simulink model "TRAMI_DCT_AT"  (R2018b)
settings: Solver=FixedStepDiscrete  StartTime=0.0  StopTime=88  FixedStep=10e-3  RelTol=1e-3  EnableMultiTasking=on
undefined symbols (not defined in the file): CONST_AP_GEAR_SUB_NEWTRAL, CONST_AP_IDLE_SPEED_CONT, CONST_AP_LOAD_SFT, CONST_AP_LOAD_SFT_HYS, CONST_CAR_WEIGHT, CONST_CL_NUM, CONST_F_DOWN_SYNCHRO, CONST_F_SYNCHRO, CONST_F_UP_SYNCHRO, CONST_FGR, CONST_I_FlYWHEEL, CONST_INATIA_CLANK, CONST_R_SHIFT_END_CD, CONST_R_SHIFT_END_EG, CONST_R_SHIFT_END_TD, CONST_R_SHIFT_END_UP, CONST_R_SYNCHRO_ENGAGE, CONST_R_TIRE, CONST_RATIO_TQ_REDUCTION, CONST_SKIP_SHIFT_MAX, CONST_SYN_NUM, CONST_T_SFT_END_EN, CONST_T_SFT_END_JUDGE, CONST_T_SFT_END_MAX, CONST_T_SFT_END_MIN, CONST_T_SHIFT_WAIT, CONST_T_TQ_PHASE_CD, CONST_T_TQ_PHASE_ND, CONST_T_TQ_PHASE_NR, CONST_T_TQ_PHASE_TD, CONST_T_TQ_PHASE_UP, CONST_TQ_CREEP_CONT, CONST_TQ_ENGAGE_CL_MARGIN, CONST_TQ_ENGAGE_CL_MIN, CONST_TQ_INATIA_TD_SHIFT, CONST_TQ_LOAD_SFT, CONST_TQ_LOAD_SFT_HYS, CONST_TQ_ND_ENGAGE, CONST_TQ_NR_ENGAGE, CONST_TQ_TQPHASE_MIN, CONST_V_IDLE_SPEED_CONT, Eng, FALSE, GrNP, GrRev, LoopTime, MAT_CL_ENGAGE, MAT_CL_SHARE_RATE, MAT_I_ACTUATOR, MAT_SYNCHRO_COM, MAT_T_GEAR_SUB_NEWTRAL, MAT_TRANS_MGR, MaxCL, Nm, PI, Shift_CD, Shift_ND, Shift_NR, Shift_TD, Shift_Up ... (+168)
libraries: simulink x26
(part 1 of 6)
settings Model: Creator=yuto-n  LastModifiedBy=yuto-n
settings DataIOCC: SaveFormat=Array  SaveOutput=off  SignalLogging=off  DSMLogging=off  SaveTime=off
settings OptimizationCC: LifeSpan=inf
settings DebuggingCC: MultiTaskRateTransMsg=warning  ParameterPrecisionLossMsg=none
settings ModelReferenceCC: PropagateSignalLabelsOutOfModel=off

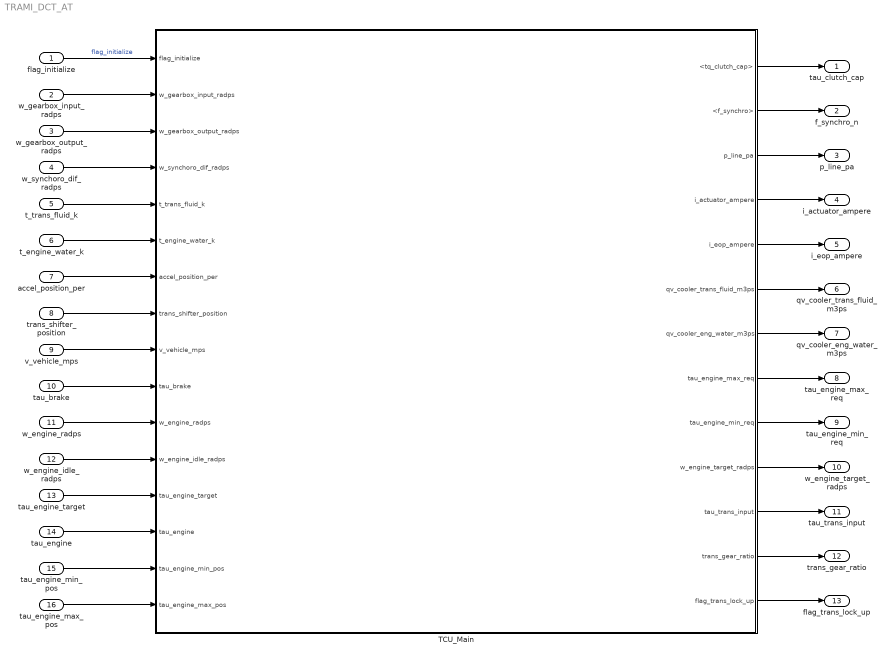
== system TRAMI_DCT_AT ==
  flag_initialize : Inport  OutDataTypeStr=boolean
      settings: AttributesFormatString=イニシャライズ要求
  w_gearbox_input_radps : Inport  Port=2  OutDataTypeStr=single
      settings: AttributesFormatString=Gearbox input speed[rad/s]
  w_gearbox_output_radps : Inport  Port=3  OutDataTypeStr=single
      settings: AttributesFormatString=Gearbox output speed[rad/s]
  w_synchoro_dif_radps : Inport  Port=4  OutDataTypeStr=single  PortDimensions=MaxSyn
      settings: AttributesFormatString=各シンクロ差回転[rad/s]
  t_trans_fluid_k : Inport  Port=5  OutDataTypeStr=single
      settings: AttributesFormatString=トランスミッション油温[K]
  t_engine_water_k : Inport  Port=6  OutDataTypeStr=single
      settings: AttributesFormatString=Eng.冷却水温[K]
  accel_position_per : Inport  Port=7  OutDataTypeStr=single
      settings: AttributesFormatString=アクセル開度[%]
  trans_shifter_position : Inport  Port=8  OutDataTypeStr=int16
      settings: AttributesFormatString=シフト位置 Rev=-1; N=0 ; D=1
  v_vehicle_mps : Inport  Port=9  OutDataTypeStr=single
      settings: AttributesFormatString=車速[m/s]
  tau_brake : Inport  Port=10  OutDataTypeStr=single
      settings: AttributesFormatString=ブレーキトルク[Nm]
  w_engine_radps : Inport  Port=11  OutDataTypeStr=single
      settings: AttributesFormatString=Engine回転[rad/s]
  w_engine_idle_radps : Inport  Port=12  OutDataTypeStr=single
      settings: AttributesFormatString=Engineアイドル回転[rad/s]
  tau_engine_target : Inport  Port=13  OutDataTypeStr=single
      settings: AttributesFormatString=Engine 目標トルク[Nm]
  tau_engine : Inport  Port=14  OutDataTypeStr=single
      settings: AttributesFormatString=Engine トルク[Nm]
  tau_engine_min_pos : Inport  Port=15  OutDataTypeStr=single
      settings: AttributesFormatString=Eng.出力可能最小トルク[Nm]
  tau_engine_max_pos : Inport  Port=16  OutDataTypeStr=single
      settings: AttributesFormatString=Eng.出力可能最小トルク[Nm]
  TCU_Main : Subsystem  TreatAsAtomicUnit=on  SystemSampleTime=0.01
      settings: AttributesFormatString=Transmission制御
  tau_clutch_cap : Outport  OutDataTypeStr=single
      settings: AttributesFormatString=各クラッチのトルク容量[Nm]
  f_synchro_n : Outport  Port=2  OutDataTypeStr=single
      settings: AttributesFormatString=各シンクロの操作力[N]
  p_line_pa : Outport  Port=3  OutDataTypeStr=single
      settings: AttributesFormatString=ライン圧[Pa]
  i_actuator_ampere : Outport  Port=4  OutDataTypeStr=single
      settings: AttributesFormatString=アクチュエータ電流[A]
  i_eop_ampere : Outport  Port=5  OutDataTypeStr=single
      settings: AttributesFormatString=電動オイルポンプ電流[A]
  qv_cooler_trans_fluid_m3ps : Outport  Port=6  OutDataTypeStr=single
      settings: AttributesFormatString=クーラーのATF流量[m3/s]
  qv_cooler_eng_water_m3ps : Outport  Port=7  OutDataTypeStr=single
      settings: AttributesFormatString=クーラーの冷却水流量[m3/s]
  tau_engine_max_req : Outport  Port=8  OutDataTypeStr=single
      settings: AttributesFormatString=エンジントルクリダクション要求[Nm]
  tau_engine_min_req : Outport  Port=9  OutDataTypeStr=single
      settings: AttributesFormatString=エンジントルクアップ要求[Nm]
  w_engine_target_radps : Outport  Port=10  OutDataTypeStr=single
      settings: AttributesFormatString=エンジン回転要求値[rad/s]
  tau_trans_input : Outport  Port=11  OutDataTypeStr=single
      settings: AttributesFormatString=トランスミッション入力軸トルク[Nm]
  trans_gear_ratio : Outport  Port=12  OutDataTypeStr=single
      settings: AttributesFormatString=ギヤ比
  flag_trans_lock_up : Outport  Port=13  OutDataTypeStr=boolean
      settings: AttributesFormatString=ロックアップ判定
  wires:
  tau_engine_max_pos/1 -> TCU_Main/16(tau_engine_max_pos)
  w_engine_idle_radps/1 -> TCU_Main/12(w_engine_idle_radps)
  accel_position_per/1 -> TCU_Main/7(accel_position_per)
  w_engine_radps/1 -> TCU_Main/11(w_engine_radps)
  tau_brake/1 -> TCU_Main/10(tau_brake)
  trans_shifter_position/1 -> TCU_Main/8(trans_shifter_position)
  t_engine_water_k/1 -> TCU_Main/6(t_engine_water_k)
  flag_initialize/1 -> TCU_Main/1(flag_initialize)  "flag_initialize"
  w_gearbox_input_radps/1 -> TCU_Main/2(w_gearbox_input_radps)
  TCU_Main/2(<f_synchro>) -> f_synchro_n/1
  TCU_Main/1(<tq_clutch_cap>) -> tau_clutch_cap/1
  tau_engine_target/1 -> TCU_Main/13(tau_engine_target)
  TCU_Main/11(tau_trans_input) -> tau_trans_input/1
  w_synchoro_dif_radps/1 -> TCU_Main/4(w_synchoro_dif_radps)
  tau_engine_min_pos/1 -> TCU_Main/15(tau_engine_min_pos)
  TCU_Main/9(tau_engine_min_req) -> tau_engine_min_req/1
  w_gearbox_output_radps/1 -> TCU_Main/3(w_gearbox_output_radps)
  TCU_Main/13(flag_trans_lock_up) -> flag_trans_lock_up/1
  TCU_Main/12(trans_gear_ratio) -> trans_gear_ratio/1
  tau_engine/1 -> TCU_Main/14(tau_engine)
  TCU_Main/4(i_actuator_ampere) -> i_actuator_ampere/1
  t_trans_fluid_k/1 -> TCU_Main/5(t_trans_fluid_k)
  v_vehicle_mps/1 -> TCU_Main/9(v_vehicle_mps)
  TCU_Main/10(w_engine_target_radps) -> w_engine_target_radps/1
  TCU_Main/3(p_line_pa) -> p_line_pa/1
  TCU_Main/6(qv_cooler_trans_fluid_m3ps) -> qv_cooler_trans_fluid_m3ps/1
  TCU_Main/7(qv_cooler_eng_water_m3ps) -> qv_cooler_eng_water_m3ps/1
  TCU_Main/5(i_eop_ampere) -> i_eop_ampere/1
  TCU_Main/8(tau_engine_max_req) -> tau_engine_max_req/1

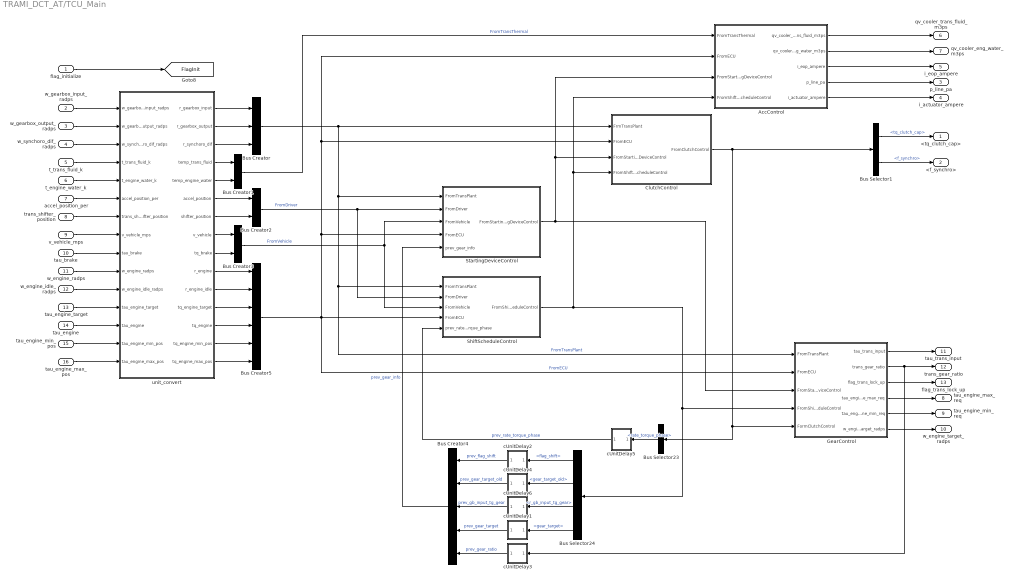
== system TRAMI_DCT_AT/TCU_Main ==
  flag_initialize : Inport
  w_gearbox_input_radps : Inport  Port=2
  w_gearbox_output_radps : Inport  Port=3
  w_synchoro_dif_radps : Inport  Port=4
  t_trans_fluid_k : Inport  Port=5
  t_engine_water_k : Inport  Port=6
  accel_position_per : Inport  Port=7
  trans_shifter_position : Inport  Port=8
  v_vehicle_mps : Inport  Port=9
  tau_brake : Inport  Port=10
  w_engine_radps : Inport  Port=11
  w_engine_idle_radps : Inport  Port=12
  tau_engine_target : Inport  Port=13
  tau_engine : Inport  Port=14
  tau_engine_min_pos : Inport  Port=15
  tau_engine_max_pos : Inport  Port=16
  AccControl : Subsystem
      settings: AttributesFormatString=BLOCK #4 油圧＆アクチュエータ制御
  Bus Creator : BusCreator  Inputs=3
  Bus Creator1 : BusCreator  Inputs=2
  Bus Creator2 : BusCreator  Inputs=2
  Bus Creator3 : BusCreator  Inputs=2
  Bus Creator4 : BusCreator  Inputs=5
  Bus Creator5 : BusCreator  Inputs=6
  Bus Selector1 : BusSelector  OutputSignals=tq_clutch_cap,f_synchro
  Bus Selector23 : BusSelector  OutputSignals=rate_torque_phase
  Bus Selector24 : BusSelector  OutputSignals=flag_shift,gear_target_old,r_gb_input_tg_gear,gear_target
  ClutchControl : Subsystem
      settings: AttributesFormatString=BLOCK #3 変速機構制御
  GearControl : Subsystem
      settings: AttributesFormatString=BLOCK #5 エンジン制御
  ShiftScheduleControl : Subsystem
      settings: AttributesFormatString=BLOCK #2 変速点制御
  StartingDeviceControl : Subsystem
      settings: AttributesFormatString="BLOCK #1  発進デバイス制御"
  cUnitDelay1 : Subsystem  mask(resetable_unit_delay){initParam=0}
      mask prompts: initParam "初期化値"
      mask Display:
      | dpoly(1,[1,0],'z')
      | text(2,10,'R')
  cUnitDelay2 : Subsystem  mask(resetable_unit_delay){initParam=0}
      mask prompts: initParam "初期化値"
      mask Display:
      | dpoly(1,[1,0],'z')
      | text(2,10,'R')
  cUnitDelay3 : Subsystem  mask(resetable_unit_delay){initParam=1}
      mask prompts: initParam "初期化値"
      mask Display:
      | dpoly(1,[1,0],'z')
      | text(2,10,'R')
  cUnitDelay4 : Subsystem  mask(resetable_unit_delay){initParam=0}
      mask prompts: initParam "初期化値"
      mask Display:
      | dpoly(1,[1,0],'z')
      | text(2,10,'R')
  cUnitDelay5 : Subsystem  mask(resetable_unit_delay){initParam=0}
      mask prompts: initParam "初期化値"
      mask Display:
      | dpoly(1,[1,0],'z')
      | text(2,10,'R')
  cUnitDelay6 : Subsystem  mask(resetable_unit_delay){initParam=0}
      mask prompts: initParam "初期化値"
      mask Display:
      | dpoly(1,[1,0],'z')
      | text(2,10,'R')
  unit_convert : Subsystem
      settings: AttributesFormatString=入力情報の単位変換
  <tq_clutch_cap> : Outport
  <f_synchro> : Outport  Port=2
  p_line_pa : Outport  Port=3
  i_actuator_ampere : Outport  Port=4
  i_eop_ampere : Outport  Port=5
  qv_cooler_trans_fluid_m3ps : Outport  Port=6
  qv_cooler_eng_water_m3ps : Outport  Port=7
  tau_engine_max_req : Outport  Port=8
  tau_engine_min_req : Outport  Port=9
  w_engine_target_radps : Outport  Port=10
  tau_trans_input : Outport  Port=11
  trans_gear_ratio : Outport  Port=12
  flag_trans_lock_up : Outport  Port=13
  tag scope: FlagInit=global
  wires:
  AccControl/2(qv_cooler_eng_water_m3ps) -> qv_cooler_eng_water_m3ps/1
  Bus Selector24/1 -> cUnitDelay2/1(<param>)  "<flag_shift>"
  Bus Selector24/2 -> cUnitDelay4/1(<param>)  "<gear_target_old>"
  cUnitDelay6/1(preParam) -> Bus Creator4/3  "prev_gb_input_tg_gear"
  AccControl/4(p_line_pa) -> p_line_pa/1
  StartingDeviceControl/1(FromStartingDeviceControl) -> GearControl/3(FromStartingDeviceControl), ClutchControl/3(FromStartingDeviceControl), AccControl/3(FromStartingDeviceControl)
  Bus Selector24/4 -> cUnitDelay1/1(<param>)  "<gear_target>"
  tau_engine_target/1 -> unit_convert/12(tau_engine_target)
  GearControl/2(trans_gear_ratio) -> trans_gear_ratio/1, cUnitDelay3/1(<param>)
  Bus Selector24/3 -> cUnitDelay6/1(<param>)  "<r_gb_input_tg_gear>"
  GearControl/4(tau_engine_max_req) -> tau_engine_max_req/1
  ShiftScheduleControl/1(FromShiftScheduleControl) -> GearControl/4(FromShiftScheduleControl), Bus Selector24/1, ClutchControl/4(FromShiftScheduleControl), AccControl/4(FromShiftScheduleControl)
  Bus Selector23/1 -> cUnitDelay5/1(<param>)  "<rate_torque_phase>"
  trans_shifter_position/1 -> unit_convert/7(trans_shifter_position)
  cUnitDelay1/1(preParam) -> Bus Creator4/4  "prev_gear_target"
  Bus Selector1/2 -> <f_synchro>/1  "<f_synchro>"
  cUnitDelay3/1(preParam) -> Bus Creator4/5  "prev_gear_ratio"
  ClutchControl/1(FromClutchControl) -> Bus Selector1/1, GearControl/5(FormClutchControl), Bus Selector23/1
  AccControl/3(i_eop_ampere) -> i_eop_ampere/1
  Bus Selector1/1 -> <tq_clutch_cap>/1  "<tq_clutch_cap>"
  cUnitDelay5/1(preParam) -> ShiftScheduleControl/5(prev_rate_torque_phase)  "prev_rate_torque_phase"
  cUnitDelay4/1(preParam) -> Bus Creator4/2  "prev_gear_target_old"
  GearControl/5(tau_engine_min_req) -> tau_engine_min_req/1
  cUnitDelay2/1(preParam) -> Bus Creator4/1  "prev_flag_shift"
  GearControl/6(w_engine_target_radps) -> w_engine_target_radps/1
  flag_initialize/1 -> [FlagInit]
  GearControl/3(flag_trans_lock_up) -> flag_trans_lock_up/1
  v_vehicle_mps/1 -> unit_convert/8(v_vehicle_mps)
  AccControl/5(i_actuator_ampere) -> i_actuator_ampere/1
  GearControl/1(tau_trans_input) -> tau_trans_input/1
  w_gearbox_output_radps/1 -> unit_convert/2(w_gearbox_output_radps)
  w_synchoro_dif_radps/1 -> unit_convert/3(w_synchoro_dif_radps)
  t_trans_fluid_k/1 -> unit_convert/4(t_trans_fluid_k)
  t_engine_water_k/1 -> unit_convert/5(t_engine_water_k)
  accel_position_per/1 -> unit_convert/6(accel_position_per)
  tau_brake/1 -> unit_convert/9(tau_brake)
  tau_engine/1 -> unit_convert/13(tau_engine)
  tau_engine_max_pos/1 -> unit_convert/15(tau_engine_max_pos)
  w_gearbox_input_radps/1 -> unit_convert/1(w_gearbox_input_radps)
  tau_engine_min_pos/1 -> unit_convert/14(tau_engine_min_pos)
  w_engine_idle_radps/1 -> unit_convert/11(w_engine_idle_radps)
  AccControl/1(qv_cooler_trans_fluid_m3ps) -> qv_cooler_trans_fluid_m3ps/1
  w_engine_radps/1 -> unit_convert/10(w_engine_radps)
  Bus Creator4/1 -> StartingDeviceControl/5(prev_gear_info)  "prev_gear_info"
  Bus Creator5/1 -> GearControl/2(FromECU), ShiftScheduleControl/4(FromECU), ClutchControl/2(FromECU), AccControl/2(FromECU), StartingDeviceControl/4(FromECU)  "FromECU"
  Bus Creator3/1 -> ShiftScheduleControl/3(FromVehicle), StartingDeviceControl/3(FromVehicle)  "FromVehicle"
  Bus Creator2/1 -> StartingDeviceControl/2(FromDriver), ShiftScheduleControl/2(FromDriver)  "FromDriver"
  Bus Creator/1 -> GearControl/1(FromTransPlant), ShiftScheduleControl/1(FromTransPlant), StartingDeviceControl/1(FromTransPlant), ClutchControl/1(FrmTransPlant)  "FromTransPlant"
  Bus Creator1/1 -> AccControl/1(FromTransThermal)  "FromTransThermal"
  unit_convert/1(r_gearbox_input) -> Bus Creator/1
  unit_convert/2(r_gearbox_output) -> Bus Creator/2
  unit_convert/3(r_synchoro_dif) -> Bus Creator/3
  unit_convert/4(temp_trans_fluid) -> Bus Creator1/1
  unit_convert/5(temp_engine_water) -> Bus Creator1/2
  unit_convert/6(accel_position) -> Bus Creator2/1
  unit_convert/7(shifter_position) -> Bus Creator2/2
  unit_convert/8(v_vehicle) -> Bus Creator3/1
  unit_convert/9(tq_brake) -> Bus Creator3/2
  unit_convert/10(r_engine) -> Bus Creator5/1
  unit_convert/11(r_engine_idle) -> Bus Creator5/2
  unit_convert/12(tq_engine_target) -> Bus Creator5/3
  unit_convert/13(tq_engine) -> Bus Creator5/4
  unit_convert/14(tq_engine_min_pos) -> Bus Creator5/5
  unit_convert/15(tq_engine_max_pos) -> Bus Creator5/6

== system TRAMI_DCT_AT/TCU_Main/AccControl ==
  FromTransThermal : Inport
  FromECU : Inport  Port=2
  FromStartingDeviceControl : Inport  Port=3
  FromShiftScheduleControl : Inport  Port=4
  AccControl : Subsystem
  Bus Selector : BusSelector  OutputSignals=temp_trans_fluid
  Bus Selector16 : BusSelector  OutputSignals=gear_target
  Bus Selector19 : BusSelector  OutputSignals=r_engine
  Bus Selector20 : BusSelector  OutputSignals=tq_gearbox_input
  qv_cooler_trans_fluid_m3ps : Outport  OutDataTypeStr=single
  qv_cooler_eng_water_m3ps : Outport  Port=2  OutDataTypeStr=single
  i_eop_ampere : Outport  Port=3  OutDataTypeStr=single
  p_line_pa : Outport  Port=4  OutDataTypeStr=single
  i_actuator_ampere : Outport  Port=5  OutDataTypeStr=single
  wires:
  FromTransThermal/1 -> Bus Selector/1
  FromECU/1 -> Bus Selector19/1
  FromStartingDeviceControl/1 -> Bus Selector20/1
  FromShiftScheduleControl/1 -> Bus Selector16/1
  Bus Selector/1 -> AccControl/1(<temp_trans_fluid>)  "<temp_trans_fluid>"
  Bus Selector19/1 -> AccControl/2(<r_engine>)  "<r_engine>"
  Bus Selector20/1 -> AccControl/3(<tq_gearbox_input>)  "<tq_gearbox_input>"
  Bus Selector16/1 -> AccControl/4(<gear_target>)  "<gear_target>"
  AccControl/1(<qv_cooler_trans_fluid_m3ps>) -> qv_cooler_trans_fluid_m3ps/1
  AccControl/2(<qv_cooler_eng_water_m3ps>) -> qv_cooler_eng_water_m3ps/1
  AccControl/3(<i_eop_ampere>) -> i_eop_ampere/1
  AccControl/4(<p_line_pa>) -> p_line_pa/1
  AccControl/5(<i_actuator_ampere>) -> i_actuator_ampere/1

== system TRAMI_DCT_AT/TCU_Main/ClutchControl ==
  FrmTransPlant : Inport
  FromECU : Inport  Port=2
  FromStartingDeviceControl : Inport  Port=3
  FromShiftScheduleControl : Inport  Port=4
  Bus Creator7 : BusCreator  Inputs=5
  Bus Selector10 : BusSelector  OutputSignals=tq_engine_target,tq_engine_min_pos
  Bus Selector22 : BusSelector  OutputSignals=flag_engine_idle_control,tq_cl_creep_cont,tq_gearbox_input,tq_cl_slip_control
  Bus Selector4 : BusSelector  OutputSignals=r_gearbox_input,r_synchoro_dif
  Bus Selector9 : BusSelector  OutputSignals=gear_target,gear_shift_kind,gear_before_shift,r_gb_input_tg_gear,gear_target_old,flag_shift,gear_sub1,gear_sub2
  ClutchControl : Subsystem
      settings: AttributesFormatString=BLOCK #3 変速機構制御
  FromClutchControl : Outport
  wires:
  Bus Creator7/1 -> FromClutchControl/1  "FromClutchControl"
  FromECU/1 -> Bus Selector10/1
  FromStartingDeviceControl/1 -> Bus Selector22/1
  FromShiftScheduleControl/1 -> Bus Selector9/1
  FrmTransPlant/1 -> Bus Selector4/1
  Bus Selector4/1 -> ClutchControl/1(<r_gearbox_input>)  "<r_gearbox_input>"
  Bus Selector4/2 -> ClutchControl/2(<r_synchoro_dif>)  "<r_synchoro_dif>"
  Bus Selector10/1 -> ClutchControl/3(<tq_engine_target>)  "<tq_engine_target>"
  Bus Selector10/2 -> ClutchControl/4(<tq_engine_min_pos>)  "<tq_engine_min_pos>"
  Bus Selector22/2 -> ClutchControl/6(<tq_cl_creep_cont>)  "<tq_cl_creep_cont>"
  Bus Selector22/3 -> ClutchControl/7(<tq_gearbox_input>)  "<tq_gearbox_input>"
  Bus Selector22/4 -> ClutchControl/8(<tq_cl_slip_control>)  "<tq_cl_slip_control>"
  Bus Selector9/1 -> ClutchControl/9(<gear_target>)  "<gear_target>"
  Bus Selector9/2 -> ClutchControl/10(<gear_shift_kind>)  "<gear_shift_kind>"
  Bus Selector9/3 -> ClutchControl/11(<gear_before_shift>)  "<gear_before_shift>"
  Bus Selector9/4 -> ClutchControl/12(<r_gb_input_tg_gear>)  "<r_gb_input_tg_gear>"
  Bus Selector9/5 -> ClutchControl/13(<gear_target_old>)  "<gear_target_old>"
  Bus Selector9/6 -> ClutchControl/14(<flag_shift>)  "<flag_shift>"
  Bus Selector9/7 -> ClutchControl/15(<gear_sub1>)  "<gear_sub1>"
  Bus Selector9/8 -> ClutchControl/16(<gear_sub2>)  "<gear_sub2>"
  ClutchControl/1(<tq_eng_shift_up_reduction>) -> Bus Creator7/1
  ClutchControl/2(<tq_inertia_engage_cl>) -> Bus Creator7/2
  ClutchControl/3(<tau_clutch_cap>) -> Bus Creator7/3
  ClutchControl/4(<rate_torque_phase>) -> Bus Creator7/4
  ClutchControl/5(<f_synchro>) -> Bus Creator7/5
  Bus Selector22/1 -> ClutchControl/5(<flag_engine_idle_control>)  "<flag_engine_idle_control>"

== system TRAMI_DCT_AT/TCU_Main/GearControl ==
  FromTransPlant : Inport
  FromECU : Inport  Port=2
  FromStartingDeviceControl : Inport  Port=3
  FromShiftScheduleControl : Inport  Port=4
  FormClutchControl : Inport  Port=5
  Bus Selector : BusSelector  OutputSignals=tq_eng_shift_up_reduction,tq_inertia_engage_cl,rate_torque_phase
  Bus Selector11 : BusSelector  OutputSignals=tq_engine_target,tq_engine_min_pos
  Bus Selector21 : BusSelector  OutputSignals=tq_torq_converter_input,tq_cl_creep_cont,tq_cl_slip_base,flag_engine_idle_control
  Bus Selector3 : BusSelector  OutputSignals=r_gearbox_input
  Bus Selector8 : BusSelector  OutputSignals=gear_target,gear_shift_kind,gear_before_shift,r_gb_input_tg_gear,flag_shift
  GearControl : Subsystem
  tau_trans_input : Outport  OutDataTypeStr=single
  trans_gear_ratio : Outport  Port=2  OutDataTypeStr=single
  flag_trans_lock_up : Outport  Port=3  OutDataTypeStr=boolean
  tau_engine_max_req : Outport  Port=4  OutDataTypeStr=single
  tau_engine_min_req : Outport  Port=5  OutDataTypeStr=single
  w_engine_target_radps : Outport  Port=6  OutDataTypeStr=single
  wires:
  FromShiftScheduleControl/1 -> Bus Selector8/1
  FromTransPlant/1 -> Bus Selector3/1
  FormClutchControl/1 -> Bus Selector/1
  FromECU/1 -> Bus Selector11/1
  FromStartingDeviceControl/1 -> Bus Selector21/1
  Bus Selector8/1 -> GearControl/8(<gear_target>)  "<gear_target>"
  Bus Selector8/2 -> GearControl/9(<gear_shift_kind>)  "<gear_shift_kind>"
  Bus Selector8/3 -> GearControl/10(<gear_before_shift>)  "<gear_before_shift>"
  Bus Selector8/4 -> GearControl/11(<r_gb_input_tg_gear>)  "<r_gb_input_tg_gear>"
  Bus Selector8/5 -> GearControl/12(<flag_shift>)  "<flag_shift>"
  Bus Selector21/1 -> GearControl/4(<tq_torq_converter_input>)  "<tq_torq_converter_input>"
  Bus Selector21/2 -> GearControl/5(<tq_cl_creep_cont>)  "<tq_cl_creep_cont>"
  Bus Selector21/3 -> GearControl/6(<tq_cl_slip_base>)  "<tq_cl_slip_base>"
  Bus Selector11/1 -> GearControl/2(<tq_engine_target>)  "<tq_engine_target>"
  Bus Selector11/2 -> GearControl/3(<tq_engine_min_pos>)  "<tq_engine_min_pos>"
  Bus Selector3/1 -> GearControl/1(<r_gearbox_input>)  "<r_gearbox_input>"
  Bus Selector/1 -> GearControl/13(<tq_eng_shift_up_reduction>)  "<tq_eng_shift_up_reduction>"
  Bus Selector/2 -> GearControl/14(<tq_inertia_engage_cl>)  "<tq_inertia_engage_cl>"
  Bus Selector/3 -> GearControl/15(<rate_torque_phase>)  "<rate_torque_phase>"
  GearControl/1(<tau_trans_input>) -> tau_trans_input/1
  GearControl/2(<trans_gear_ratio>) -> trans_gear_ratio/1
  GearControl/3(<flag_trans_lock_up>) -> flag_trans_lock_up/1
  GearControl/4(<tau_engine_max_req>) -> tau_engine_max_req/1
  GearControl/5(<tau_engine_min_req>) -> tau_engine_min_req/1
  GearControl/6(<w_engine_target_radps>) -> w_engine_target_radps/1
  Bus Selector21/4 -> GearControl/7(<flag_engine_idle_control>)  "<flag_engine_idle_control>"

== system TRAMI_DCT_AT/TCU_Main/ShiftScheduleControl ==
  FromTransPlant : Inport
  FromDriver : Inport  Port=2
  FromVehicle : Inport  Port=3
  FromECU : Inport  Port=4
  prev_rate_torque_phase : Inport  Port=5  OutDataTypeStr=single
  Bus Creator6 : BusCreator  Inputs=8
  Bus Selector1 : BusSelector  OutputSignals=r_gearbox_output,r_gearbox_input
  Bus Selector13 : BusSelector  OutputSignals=tq_engine_target
  Bus Selector15 : BusSelector  OutputSignals=v_vehicle
  Bus Selector2 : BusSelector  OutputSignals=accel_position,shifter_position
  ShiftScheduleControl : Subsystem
      settings: AttributesFormatString=BLOCK #2 変速点制御
  FromShiftScheduleControl : Outport
  wires:
  FromECU/1 -> Bus Selector13/1
  FromDriver/1 -> Bus Selector2/1
  FromVehicle/1 -> Bus Selector15/1
  FromTransPlant/1 -> Bus Selector1/1
  Bus Creator6/1 -> FromShiftScheduleControl/1  "FromShiftScheduleControl"
  Bus Selector1/1 -> ShiftScheduleControl/1(<r_gearbox_output>)  "<r_gearbox_output>"
  Bus Selector1/2 -> ShiftScheduleControl/2(<r_gearbox_input>)  "<r_gearbox_input>"
  Bus Selector13/1 -> ShiftScheduleControl/6(<tq_engine_target>)  "<tq_engine_target>"
  Bus Selector2/1 -> ShiftScheduleControl/3(<accel_position>)  "<accel_position>"
  Bus Selector2/2 -> ShiftScheduleControl/4(<shifter_position>)  "<shifter_position>"
  Bus Selector15/1 -> ShiftScheduleControl/5(<v_vehicle>)  "<v_vehicle>"
  prev_rate_torque_phase/1 -> ShiftScheduleControl/7(<rate_torque_phase>)
  ShiftScheduleControl/1(<gear_shift_kind>) -> Bus Creator6/1
  ShiftScheduleControl/2(<gear_target>) -> Bus Creator6/2
  ShiftScheduleControl/3(<gear_target_old>) -> Bus Creator6/3
  ShiftScheduleControl/4(<gear_before_shift>) -> Bus Creator6/4
  ShiftScheduleControl/5(<r_gb_input_tg_gear>) -> Bus Creator6/5
  ShiftScheduleControl/6(<flag_shift>) -> Bus Creator6/6
  ShiftScheduleControl/7(<gear_sub1>) -> Bus Creator6/7
  ShiftScheduleControl/8(<gear_sub2>) -> Bus Creator6/8

== system TRAMI_DCT_AT/TCU_Main/StartingDeviceControl ==
  FromTransPlant : Inport
  FromDriver : Inport  Port=2
  FromVehicle : Inport  Port=3
  FromECU : Inport  Port=4
  prev_gear_info : Inport  Port=5
  Bus Creator5 : BusCreator  Inputs=6
  Bus Selector1 : BusSelector  OutputSignals=v_vehicle
  Bus Selector12 : BusSelector  OutputSignals=r_engine,tq_engine_target,r_engine_idle
  Bus Selector2 : BusSelector  OutputSignals=r_gearbox_input
  Bus Selector3 : BusSelector  OutputSignals=prev_gear_ratio,prev_gear_target,prev_gb_input_tg_gear,prev_gear_target_old,prev_flag_shift
  Bus Selector4 : BusSelector  OutputSignals=accel_position
  StartingDeviceControl : Subsystem
      settings: AttributesFormatString="BLOCK #1  発進デバイス制御"
  FromStartingDeviceControl : Outport
  wires:
  FromECU/1 -> Bus Selector12/1
  FromTransPlant/1 -> Bus Selector2/1
  Bus Creator5/1 -> FromStartingDeviceControl/1  "FromStartingDeviceControl"
  Bus Selector2/1 -> StartingDeviceControl/1(<r_gearbox_input>)  "<r_gearbox_input>"
  Bus Selector12/1 -> StartingDeviceControl/4(<r_engine>)  "<r_engine>"
  Bus Selector12/2 -> StartingDeviceControl/5(<tq_engine_target>)  "<tq_engine_target>"
  Bus Selector12/3 -> StartingDeviceControl/6(<r_engine_idle>)  "<r_engine_idle>"
  StartingDeviceControl/1(<tq_cl_creep_cont>) -> Bus Creator5/1
  StartingDeviceControl/2(<tq_torq_converter_input>) -> Bus Creator5/2
  StartingDeviceControl/3(<tq_gearbox_input>) -> Bus Creator5/3
  StartingDeviceControl/4(<tq_cl_slip_control>) -> Bus Creator5/4
  StartingDeviceControl/5(<tq_cl_slip_base>) -> Bus Creator5/5
  prev_gear_info/1 -> Bus Selector3/1
  FromVehicle/1 -> Bus Selector1/1
  FromDriver/1 -> Bus Selector4/1
  Bus Selector4/1 -> StartingDeviceControl/2(<accel_position>)  "<accel_position>"
  Bus Selector1/1 -> StartingDeviceControl/3(<v_vehicle>)  "<v_vehicle>"
  StartingDeviceControl/6(flag_engine_idle_control) -> Bus Creator5/6
  Bus Selector3/1 -> StartingDeviceControl/7(<gear_ratio>)  "<prev_gear_ratio>"
  Bus Selector3/2 -> StartingDeviceControl/8(<gear_target>)  "<prev_gear_target>"
  Bus Selector3/3 -> StartingDeviceControl/9(<r_gb_input_tg_gear>)  "<prev_gb_input_tg_gear>"
  Bus Selector3/4 -> StartingDeviceControl/10(<gear_target_old>)  "<prev_gear_target_old>"
  Bus Selector3/5 -> StartingDeviceControl/11(<flag_shift>)  "<prev_flag_shift>"

== system TRAMI_DCT_AT/TCU_Main/cUnitDelay1 ==
  <param> : Inport
  Constant13 : Constant  Value=initParam  OutDataTypeStr=single
  Switch12 : Switch  Criteria=u2 > Threshold
  Unit Delay2 : UnitDelay  InitialCondition=zeros(size(initParam))  SampleTime=-1
  preParam : Outport
  wires:
  <param>/1 -> Unit Delay2/1
  Constant13/1 -> Switch12/1
  [FlagInit] -> Switch12/2
  Switch12/1 -> preParam/1
  Unit Delay2/1 -> Switch12/3

== system TRAMI_DCT_AT/TCU_Main/cUnitDelay2 ==
  <param> : Inport
  Constant13 : Constant  Value=initParam  OutDataTypeStr=single
  Switch12 : Switch  Criteria=u2 > Threshold
  Unit Delay2 : UnitDelay  InitialCondition=zeros(size(initParam))  SampleTime=-1
  preParam : Outport
  wires:
  Unit Delay2/1 -> Switch12/3
  Switch12/1 -> preParam/1
  [FlagInit] -> Switch12/2
  Constant13/1 -> Switch12/1
  <param>/1 -> Unit Delay2/1

== system TRAMI_DCT_AT/TCU_Main/cUnitDelay3 ==
  <param> : Inport
  Constant13 : Constant  Value=initParam  OutDataTypeStr=single
  Switch12 : Switch  Criteria=u2 > Threshold
  Unit Delay2 : UnitDelay  InitialCondition=zeros(size(initParam))  SampleTime=-1
  preParam : Outport
  wires:
  <param>/1 -> Unit Delay2/1
  Constant13/1 -> Switch12/1
  [FlagInit] -> Switch12/2
  Switch12/1 -> preParam/1
  Unit Delay2/1 -> Switch12/3

== system TRAMI_DCT_AT/TCU_Main/cUnitDelay4 ==
  <param> : Inport
  Constant13 : Constant  Value=initParam  OutDataTypeStr=single
  Switch12 : Switch  Criteria=u2 > Threshold
  Unit Delay2 : UnitDelay  InitialCondition=zeros(size(initParam))  SampleTime=-1
  preParam : Outport
  wires:
  <param>/1 -> Unit Delay2/1
  Constant13/1 -> Switch12/1
  [FlagInit] -> Switch12/2
  Switch12/1 -> preParam/1
  Unit Delay2/1 -> Switch12/3

== system TRAMI_DCT_AT/TCU_Main/cUnitDelay5 ==
  <param> : Inport
  Constant13 : Constant  Value=initParam  OutDataTypeStr=single
  Switch12 : Switch  Criteria=u2 > Threshold
  Unit Delay2 : UnitDelay  InitialCondition=zeros(size(initParam))  SampleTime=-1
  preParam : Outport
  wires:
  Unit Delay2/1 -> Switch12/3
  Switch12/1 -> preParam/1
  [FlagInit] -> Switch12/2
  Constant13/1 -> Switch12/1
  <param>/1 -> Unit Delay2/1

== system TRAMI_DCT_AT/TCU_Main/cUnitDelay6 ==
  <param> : Inport
  Constant13 : Constant  Value=initParam  OutDataTypeStr=single
  Switch12 : Switch  Criteria=u2 > Threshold
  Unit Delay2 : UnitDelay  InitialCondition=zeros(size(initParam))  SampleTime=-1
  preParam : Outport
  wires:
  Unit Delay2/1 -> Switch12/3
  Switch12/1 -> preParam/1
  [FlagInit] -> Switch12/2
  Constant13/1 -> Switch12/1
  <param>/1 -> Unit Delay2/1

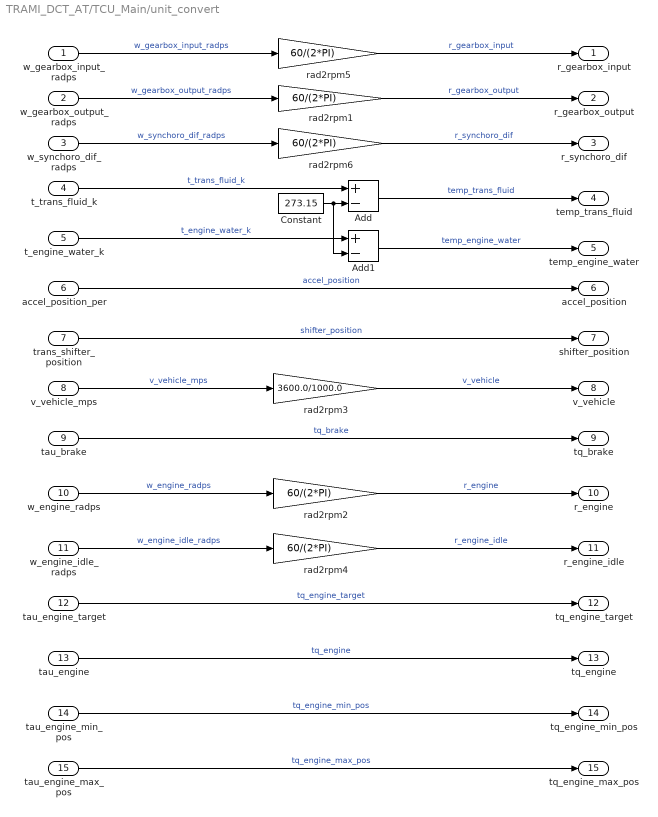
== system TRAMI_DCT_AT/TCU_Main/unit_convert ==
  w_gearbox_input_radps : Inport  OutDataTypeStr=single
  w_gearbox_output_radps : Inport  Port=2  OutDataTypeStr=single
  w_synchoro_dif_radps : Inport  Port=3  OutDataTypeStr=single
  t_trans_fluid_k : Inport  Port=4  OutDataTypeStr=single
  t_engine_water_k : Inport  Port=5  OutDataTypeStr=single
  accel_position_per : Inport  Port=6  OutDataTypeStr=single
  trans_shifter_position : Inport  Port=7  OutDataTypeStr=int16
  v_vehicle_mps : Inport  Port=8  OutDataTypeStr=single
  tau_brake : Inport  Port=9  OutDataTypeStr=single
  w_engine_radps : Inport  Port=10  OutDataTypeStr=single
  w_engine_idle_radps : Inport  Port=11  OutDataTypeStr=single
  tau_engine_target : Inport  Port=12  OutDataTypeStr=single
  tau_engine : Inport  Port=13  OutDataTypeStr=single
  tau_engine_min_pos : Inport  Port=14  OutDataTypeStr=single
  tau_engine_max_pos : Inport  Port=15  OutDataTypeStr=single
  Add : Sum  Inputs=+-  OutDataTypeStr=single
      settings: AttributesFormatString=K->℃
  Add1 : Sum  Inputs=+-  OutDataTypeStr=single
      settings: AttributesFormatString=K->℃
  Constant : Constant  Value=273.15  OutDataTypeStr=single
  rad2rpm{1..2,4..6} (5 alike) : Gain  Gain=60/(2*PI)  OutDataTypeStr=single
      settings: AttributesFormatString=rad/s->rpm
  rad2rpm3 : Gain  Gain=3600.0/1000.0  OutDataTypeStr=single
      settings: AttributesFormatString=m/s->km/h
  r_gearbox_input : Outport  OutDataTypeStr=single
  r_gearbox_output : Outport  Port=2  OutDataTypeStr=single
  r_synchoro_dif : Outport  Port=3  OutDataTypeStr=single
  temp_trans_fluid : Outport  Port=4  OutDataTypeStr=single
  temp_engine_water : Outport  Port=5  OutDataTypeStr=single
  accel_position : Outport  Port=6  OutDataTypeStr=single
  shifter_position : Outport  Port=7  OutDataTypeStr=int16
  v_vehicle : Outport  Port=8  OutDataTypeStr=single
  tq_brake : Outport  Port=9  OutDataTypeStr=single
  r_engine : Outport  Port=10  OutDataTypeStr=single
  r_engine_idle : Outport  Port=11  OutDataTypeStr=single
  tq_engine_target : Outport  Port=12  OutDataTypeStr=single
  tq_engine : Outport  Port=13  OutDataTypeStr=single
  tq_engine_min_pos : Outport  Port=14  OutDataTypeStr=single
  tq_engine_max_pos : Outport  Port=15  OutDataTypeStr=single
  wires:
  w_gearbox_output_radps/1 -> rad2rpm1/1  "w_gearbox_output_radps"
  Add/1 -> temp_trans_fluid/1  "temp_trans_fluid"
  Constant/1 -> Add1/2, Add/2
  accel_position_per/1 -> accel_position/1  "accel_position"
  tau_engine_max_pos/1 -> tq_engine_max_pos/1  "tq_engine_max_pos"
  tau_engine_target/1 -> tq_engine_target/1  "tq_engine_target"
  w_gearbox_input_radps/1 -> rad2rpm5/1  "w_gearbox_input_radps"
  rad2rpm2/1 -> r_engine/1  "r_engine"
  w_engine_radps/1 -> rad2rpm2/1  "w_engine_radps"
  w_synchoro_dif_radps/1 -> rad2rpm6/1  "w_synchoro_dif_radps"
  rad2rpm1/1 -> r_gearbox_output/1  "r_gearbox_output"
  trans_shifter_position/1 -> shifter_position/1  "shifter_position"
  rad2rpm4/1 -> r_engine_idle/1  "r_engine_idle"
  t_trans_fluid_k/1 -> Add/1  "t_trans_fluid_k"
  w_engine_idle_radps/1 -> rad2rpm4/1  "w_engine_idle_radps"
  t_engine_water_k/1 -> Add1/1  "t_engine_water_k"
  rad2rpm6/1 -> r_synchoro_dif/1  "r_synchoro_dif"
  Add1/1 -> temp_engine_water/1  "temp_engine_water"
  rad2rpm5/1 -> r_gearbox_input/1  "r_gearbox_input"
  v_vehicle_mps/1 -> rad2rpm3/1  "v_vehicle_mps"
  rad2rpm3/1 -> v_vehicle/1  "v_vehicle"
  tau_engine/1 -> tq_engine/1  "tq_engine"
  tau_engine_min_pos/1 -> tq_engine_min_pos/1  "tq_engine_min_pos"
  tau_brake/1 -> tq_brake/1  "tq_brake"

== system TRAMI_DCT_AT/TCU_Main/AccControl/AccControl ==
  <temp_trans_fluid> : Inport  OutDataTypeStr=single
  <r_engine> : Inport  Port=2  OutDataTypeStr=single
  <tq_gearbox_input> : Inport  Port=3  OutDataTypeStr=single
  <gear_target> : Inport  Port=4  OutDataTypeStr=int16
  Gain1 : Gain  Gain=1000.0  OutDataTypeStr=single
  Gain2 : Gain  Gain=1/1000.0  OutDataTypeStr=single
  Gain3 : Gain  Gain=1/60.0  OutDataTypeStr=single
  Gain4 : Gain  Gain=1/1000.0  OutDataTypeStr=single
  Gain5 : Gain  Gain=1/60.0  OutDataTypeStr=single
  TCU_Acutuator_Control : Subsystem
      settings: AttributesFormatString=トランスミッションアクチュエータ電流制御
  TCU_Cooler_Flow_Rate_Control : Subsystem
      settings: AttributesFormatString=クーラー流量制御
  TCU_EOP_Control : Subsystem
      settings: AttributesFormatString=電動オイルポンプ制御
  TCU_Pressure_Line_Control : Subsystem
      settings: AttributesFormatString=ライン圧制御
  <qv_cooler_trans_fluid_m3ps> : Outport  OutDataTypeStr=single
  <qv_cooler_eng_water_m3ps> : Outport  Port=2  OutDataTypeStr=single
  <i_eop_ampere> : Outport  Port=3  OutDataTypeStr=single
  <p_line_pa> : Outport  Port=4  OutDataTypeStr=single
  <i_actuator_ampere> : Outport  Port=5  OutDataTypeStr=single
  wires:
  TCU_Cooler_Flow_Rate_Control/2(q_cooler_engine_water) -> Gain4/1
  Gain3/1 -> <qv_cooler_trans_fluid_m3ps>/1  "qv_cooler_trans_fluid_m3ps"
  TCU_Acutuator_Control/1(i_actuator) -> <i_actuator_ampere>/1
  TCU_Cooler_Flow_Rate_Control/1(q_cooler_trans_fluid) -> Gain2/1
  TCU_EOP_Control/1(i_eop) -> <i_eop_ampere>/1
  Gain5/1 -> <qv_cooler_eng_water_m3ps>/1  "qv_cooler_eng_water_m3ps"
  <tq_gearbox_input>/1 -> TCU_Pressure_Line_Control/1(tq_gearbox_input)
  TCU_Pressure_Line_Control/1(p_line) -> Gain1/1
  Gain4/1 -> Gain5/1
  Gain1/1 -> <p_line_pa>/1  "p_line_pa"
  <gear_target>/1 -> TCU_Acutuator_Control/1(gear_target), TCU_Pressure_Line_Control/2(gear_target)
  Gain2/1 -> Gain3/1
  <temp_trans_fluid>/1 -> TCU_EOP_Control/1(temp_trans_fluid), TCU_Cooler_Flow_Rate_Control/1(temp_trans_fluid)
  <r_engine>/1 -> TCU_EOP_Control/2(r_engine)

== system TRAMI_DCT_AT/TCU_Main/ClutchControl/ClutchControl ==
  <r_gearbox_input> : Inport  OutDataTypeStr=single
  <r_synchoro_dif> : Inport  Port=2  OutDataTypeStr=single
  <tq_engine_target> : Inport  Port=3  OutDataTypeStr=single
  <tq_engine_min_pos> : Inport  Port=4  OutDataTypeStr=single
  <flag_engine_idle_control> : Inport  Port=5  OutDataTypeStr=boolean
  <tq_cl_creep_cont> : Inport  Port=6  OutDataTypeStr=single
  <tq_gearbox_input> : Inport  Port=7  OutDataTypeStr=single
  <tq_cl_slip_control> : Inport  Port=8  OutDataTypeStr=single
  <gear_target> : Inport  Port=9  OutDataTypeStr=int16
  <gear_shift_kind> : Inport  Port=10  OutDataTypeStr=int16
  <gear_before_shift> : Inport  Port=11  OutDataTypeStr=int16
  <r_gb_input_tg_gear> : Inport  Port=12  OutDataTypeStr=single
  <gear_target_old> : Inport  Port=13  OutDataTypeStr=int16
  <flag_shift> : Inport  Port=14  OutDataTypeStr=boolean
  <gear_sub1> : Inport  Port=15  OutDataTypeStr=int16
  <gear_sub2> : Inport  Port=16  OutDataTypeStr=int16
  TCU_Clutch_Control : Subsystem  VariantControl=CONST_SYN_NUM == 0
      settings: AttributesFormatString=各クラッチ容量の計算（分担トルク未考慮）
  TCU_Clutch_Torque_Capacity : Subsystem  VariantControl=CONST_SYN_NUM == 0
      settings: AttributesFormatString=各クラッチの分担トルクを掛けて、クラッチ容量を求める。
  TCU_Gear_Clutch_Control : Subsystem
      settings: AttributesFormatString=clutch制御用ギヤ段 (TorqPhase前で切り替わる)の算出
  TCU_SYNCHORO_CONTROL_AT_DCT : Subsystem  Variant=on
      settings: AttributesFormatString=シンクロ制御
  TCU_SYNCHORO_STATUS_AT_DCT : Subsystem  Variant=on
      settings: AttributesFormatString=シンクロ同期判定
  TCU_Shift_Clutch : Subsystem
      settings: AttributesFormatString=締結・解放クラッチの算出
  TCU_Shift_Inertia_Torq : Subsystem
      settings: AttributesFormatString=変速時のイナーシャトルクの算出
  TCU_Torque_Phase : Subsystem
      settings: AttributesFormatString=トルクフェイズの移行比率の算出
  Terminator{1..3,28..32} (8 alike) : Terminator
  cUnitDelay1 : Subsystem  mask(resetable_unit_delay){initParam=0}
      mask prompts: initParam "初期化値"
      mask Display:
      | dpoly(1,[1,0],'z')
      | text(2,10,'R')
  cUnitDelay3 : Subsystem  mask(resetable_unit_delay){initParam=0}
      mask prompts: initParam "初期化値"
      mask Display:
      | dpoly(1,[1,0],'z')
      | text(2,10,'R')
  <tq_eng_shift_up_reduction> : Outport  OutDataTypeStr=single
  <tq_inertia_engage_cl> : Outport  Port=2  OutDataTypeStr=single
  <tau_clutch_cap> : Outport  Port=3  OutDataTypeStr=single
  <rate_torque_phase> : Outport  Port=4  OutDataTypeStr=single
  <f_synchro> : Outport  Port=5  OutDataTypeStr=single
  wires:
  <gear_target>/1 -> TCU_SYNCHORO_STATUS_AT_DCT/1(gear_target), TCU_SYNCHORO_CONTROL_AT_DCT/1(gear_target), TCU_Gear_Clutch_Control/2(gear_target), TCU_Torque_Phase/4(gear_target), TCU_Clutch_Control/10(gear_target), TCU_Shift_Clutch/1(gear_target), TCU_Shift_Inertia_Torq/2(gear_target), TCU_Clutch_Torque_Capacity/1(gear_target)
  <flag_shift>/1 -> TCU_Clutch_Control/6(flag_shift), TCU_Torque_Phase/1(flag_shift)
  TCU_Shift_Inertia_Torq/2(tq_inertia_release_cl) -> TCU_Clutch_Control/4(tq_inertia_release_cl)
  <r_gb_input_tg_gear>/1 -> TCU_Gear_Clutch_Control/6(r_gb_input_tg_gear), TCU_Shift_Inertia_Torq/5(r_gb_input_tg_gear)
  TCU_Shift_Inertia_Torq/1(tq_inertia_engage_cl) -> TCU_Clutch_Control/3(tq_inertia_engage_cl), <tq_inertia_engage_cl>/1
  TCU_SYNCHORO_STATUS_AT_DCT/1(flag_synchro_ready) -> TCU_Gear_Clutch_Control/1(flag_synchro_ready)
  <gear_before_shift>/1 -> TCU_SYNCHORO_CONTROL_AT_DCT/2(gear_before_shift), TCU_Gear_Clutch_Control/3(gear_before_shift), TCU_Shift_Clutch/2(gear_before_shift), TCU_Clutch_Torque_Capacity/2(gear_before_shift)
  TCU_Shift_Clutch/1(n_engage_clutch) -> TCU_Clutch_Control/7(n_engage_clutch)
  <r_gearbox_input>/1 -> TCU_Gear_Clutch_Control/5(r_gearbox_input), TCU_Shift_Inertia_Torq/4(r_gearbox_input)
  TCU_Clutch_Torque_Capacity/2(rate_clutch_share) -> Terminator1/1
  <gear_shift_kind>/1 -> TCU_Gear_Clutch_Control/4(gear_shift_kind), TCU_Torque_Phase/2(gear_shift_kind), TCU_Shift_Inertia_Torq/1(gear_shift_kind)
  TCU_Shift_Inertia_Torq/6(tq_inertia) -> Terminator3/1
  TCU_Shift_Clutch/2(n_release_clutch) -> TCU_Clutch_Control/8(n_release_clutch)
  TCU_Shift_Inertia_Torq/3(tq_eng_shift_up_reduction) -> <tq_eng_shift_up_reduction>/1
  TCU_Clutch_Control/2(tq_engage_cl_cap) -> Terminator28/1
  TCU_Gear_Clutch_Control/1(gear_cl_com) -> TCU_Torque_Phase/3(gear_cl_com), TCU_Clutch_Control/9(gear_cl_com)
  TCU_Shift_Inertia_Torq/4(t_shift_time_tg) -> Terminator29/1
  TCU_SYNCHORO_CONTROL_AT_DCT/2(flag_synchro_com) -> Terminator2/1
  TCU_Clutch_Control/3(tq_release_cl_cap) -> Terminator30/1
  TCU_Torque_Phase/1(rate_torque_phase) -> <rate_torque_phase>/1, TCU_Clutch_Control/5(rate_torque_phase)
  TCU_Shift_Inertia_Torq/5(r_delta_speed) -> Terminator31/1
  TCU_Clutch_Control/1(tq_clutch_cap_inp) -> TCU_Clutch_Torque_Capacity/3(tq_clutch_cap_inp)
  <gear_sub1>/1 -> TCU_SYNCHORO_CONTROL_AT_DCT/3(gear_sub1)
  <gear_target_old>/1 -> TCU_Shift_Inertia_Torq/3(gear_target_old)
  <tq_cl_creep_cont>/1 -> TCU_Clutch_Control/12(tq_cl_creep_cont)
  <r_synchoro_dif>/1 -> TCU_SYNCHORO_STATUS_AT_DCT/3(r_synchoro_dif)
  <tq_engine_target>/1 -> TCU_Shift_Inertia_Torq/6(tq_engine_target)
  <tq_cl_slip_control>/1 -> TCU_Clutch_Control/2(tq_cl_slip_control)
  <tq_gearbox_input>/1 -> TCU_Clutch_Control/1(tq_gearbox_input)
  TCU_Clutch_Torque_Capacity/1(tq_clutch_cap) -> <tau_clutch_cap>/1
  <gear_sub2>/1 -> TCU_SYNCHORO_CONTROL_AT_DCT/4(gear_sub2)
  <tq_engine_min_pos>/1 -> TCU_Shift_Inertia_Torq/7(tq_engine_min_pos)
  <flag_engine_idle_control>/1 -> TCU_Clutch_Control/11(flag_engine_idle_control)
  TCU_Torque_Phase/2(t_tq_phase) -> Terminator32/1, cUnitDelay3/1(<param>)
  cUnitDelay3/1(preParam) -> TCU_Torque_Phase/5(t_tq_phase_old)
  TCU_SYNCHORO_CONTROL_AT_DCT/1(f_synchro) -> <f_synchro>/1, cUnitDelay1/1(<param>)  "f_synchro"
  cUnitDelay1/1(preParam) -> TCU_SYNCHORO_CONTROL_AT_DCT/5(f_synchro_old), TCU_SYNCHORO_STATUS_AT_DCT/2(f_synchro)  "f_synchro_OLD"

== system TRAMI_DCT_AT/TCU_Main/GearControl/GearControl ==
  <r_gearbox_input> : Inport  OutDataTypeStr=single
  <tq_engine_target> : Inport  Port=2  OutDataTypeStr=single
  <tq_engine_min_pos> : Inport  Port=3  OutDataTypeStr=single
  <tq_torq_converter_input> : Inport  Port=4  OutDataTypeStr=single
  <tq_cl_creep_cont> : Inport  Port=5  OutDataTypeStr=single
  <tq_cl_slip_base> : Inport  Port=6  OutDataTypeStr=single
  <flag_engine_idle_control> : Inport  Port=7  OutDataTypeStr=boolean
  <gear_target> : Inport  Port=8  OutDataTypeStr=int16
  <gear_shift_kind> : Inport  Port=9  OutDataTypeStr=int16
  <gear_before_shift> : Inport  Port=10  OutDataTypeStr=int16
  <r_gb_input_tg_gear> : Inport  Port=11  OutDataTypeStr=single
  <flag_shift> : Inport  Port=12  OutDataTypeStr=boolean
  <tq_eng_shift_up_reduction> : Inport  Port=13  OutDataTypeStr=single
  <tq_inertia_engage_cl> : Inport  Port=14  OutDataTypeStr=single
  <rate_torque_phase> : Inport  Port=15  OutDataTypeStr=single
  Gain : Gain  Gain=(2*pi)/60.0  OutDataTypeStr=single
  TCU_Engine_Torque_Request : Subsystem
      settings: AttributesFormatString=エンジントルク制御要求(各制御のトルク要求を調停する)
  TCU_Information_For_ECU : Subsystem
      settings: AttributesFormatString=ECUのための制御
  TCU_Up_Shift_Torque_Reduction : Subsystem
      settings: AttributesFormatString=UpShift時のトルクリダクション
  <tau_trans_input> : Outport  OutDataTypeStr=single
  <trans_gear_ratio> : Outport  Port=2  OutDataTypeStr=single
  <flag_trans_lock_up> : Outport  Port=3  OutDataTypeStr=boolean
  <tau_engine_max_req> : Outport  Port=4  OutDataTypeStr=single
  <tau_engine_min_req> : Outport  Port=5  OutDataTypeStr=single
  <w_engine_target_radps> : Outport  Port=6  OutDataTypeStr=single
  wires:
  TCU_Information_For_ECU/1(tq_trans_input) -> <tau_trans_input>/1
  TCU_Up_Shift_Torque_Reduction/1(tq_shift_up_target) -> TCU_Engine_Torque_Request/1(tq_shift_up_target)
  <flag_engine_idle_control>/1 -> TCU_Information_For_ECU/2(flag_engine_idle_control)  "flag_engine_idle_control"
  <tq_engine_target>/1 -> TCU_Up_Shift_Torque_Reduction/9(tq_engine_target)
  TCU_Up_Shift_Torque_Reduction/2(flag_shift_up_tq_request) -> TCU_Engine_Torque_Request/2(flag_shift_up_tq_request)
  TCU_Engine_Torque_Request/2(tq_engine_min_req) -> <tau_engine_min_req>/1
  TCU_Information_For_ECU/2(gear_ratio) -> <trans_gear_ratio>/1
  TCU_Engine_Torque_Request/3(r_engine_target) -> Gain/1
  TCU_Information_For_ECU/3(flag_lock_up) -> <flag_trans_lock_up>/1
  <gear_target>/1 -> TCU_Information_For_ECU/1(gear_target), TCU_Up_Shift_Torque_Reduction/3(gear_target)
  TCU_Engine_Torque_Request/1(tq_engine_max_req) -> <tau_engine_max_req>/1
  <flag_shift>/1 -> TCU_Up_Shift_Torque_Reduction/5(flag_shift)
  Gain/1 -> <w_engine_target_radps>/1  "w_engine_target_radps"
  <tq_torq_converter_input>/1 -> TCU_Information_For_ECU/3(tq_torq_converter_input)
  <tq_inertia_engage_cl>/1 -> TCU_Up_Shift_Torque_Reduction/11(tq_inertia_engage_cl)
  <r_gearbox_input>/1 -> TCU_Up_Shift_Torque_Reduction/8(r_gearbox_input)
  <tq_engine_min_pos>/1 -> TCU_Up_Shift_Torque_Reduction/10(tq_engine_min_pos)
  <tq_cl_creep_cont>/1 -> TCU_Information_For_ECU/4(tq_cl_creep_cont)
  <gear_shift_kind>/1 -> TCU_Up_Shift_Torque_Reduction/2(gear_shift_kind)
  <rate_torque_phase>/1 -> TCU_Up_Shift_Torque_Reduction/6(rate_torque_phase)
  <r_gb_input_tg_gear>/1 -> TCU_Up_Shift_Torque_Reduction/7(r_gb_input_tg_gear)
  <tq_cl_slip_base>/1 -> TCU_Information_For_ECU/5(tq_cl_slip_base)
  <tq_eng_shift_up_reduction>/1 -> TCU_Up_Shift_Torque_Reduction/1(tq_eng_shift_up_reduction)
  <gear_before_shift>/1 -> TCU_Up_Shift_Torque_Reduction/4(gear_before_shift)
